simulink model "autopilot_gazebo"  (R2016a)
settings: Solver=ode3  StartTime=0.0  StopTime=30  FixedStep=0.01  RelTol=1e-3
values from neighbouring files (symbols this model uses):
  Kx = KK(:,1:8)    [drone_config.m]
  Ky = KK(:,9:12)    [drone_config.m]
undefined symbols (not defined in the file or in its folder): DiscIntNeverNeededParam, sigbuilder_block, W, X, Y, Z
libraries: simulink_extras x3, robotlib x3, aerolibtransform2 x2, simulink x1
settings Model: Creator=rcasado  LastModifiedBy=rcasado
settings DataIOCC: LimitDataPoints=on  SaveFormat=Array
settings DebuggingCC: MultiTaskRateTransMsg=warning  AllowSymbolicDim=off
settings HardwareCC: ProdBitPerPointer=32  ProdLargestAtomicFloat=None  ProdIntDivRoundTo=Undefined  ProdEndianess=Unspecified  ProdWordSize=32  ProdHWDeviceType=32-bit Generic
settings ModelReferenceCC: PropagateSignalLabelsOutOfModel=off
settings ConfigComp: CovModelRefEnable=Off

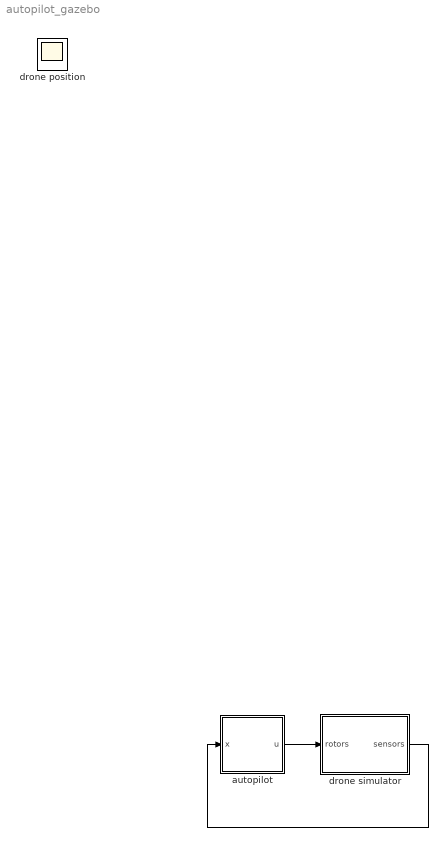
== system autopilot_gazebo ==
  autopilot : Stateflow chart  TreatAsAtomicUnit=on
  drone simulator : Subsystem
  drone position : Scope
  wires:
  drone simulator/1(sensors) -> autopilot/1(x)
  autopilot/1(u) -> drone simulator/1(rotors)

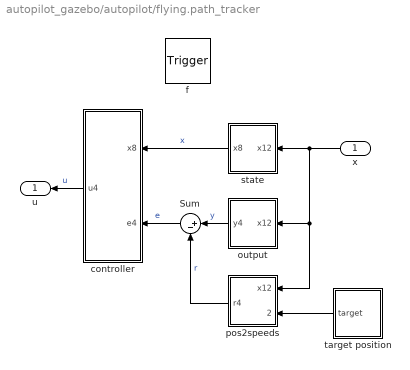
== system autopilot_gazebo/autopilot/flying.path_tracker ==
  x : Inport  OutDataTypeStr=double  PortDimensions=12
  f : TriggerPort  TriggerType=function-call  VariantControl=Variant
      settings: CopyFcn=Stateflow.SLINSF.SimulinkMan.removeBlockPreDeleteFcn  PreDeleteFcn=Stateflow.SLINSF.SimulinkMan.unsafePredeleteFcn
  Sum : Sum  Inputs=|+-
  controller : Subsystem
  output : Subsystem
  pos2speeds : Subsystem
  state : Subsystem
  target position : Subsystem
  u : Outport
  wires:
  x/1 -> pos2speeds/1(x12), output/1(x12), state/1(x12)
  pos2speeds/1(r4) -> Sum/2  "r"
  controller/1(u4) -> u/1  "u"
  output/1(y4) -> Sum/1  "y"
  state/1(x8) -> controller/1(x8)  "x"
  Sum/1 -> controller/2(e4)  "e"
  target position/1(target) -> pos2speeds/2(target)

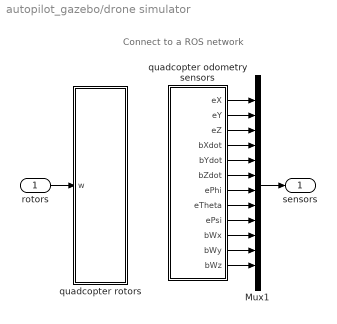
== system autopilot_gazebo/drone simulator ==
  note: Connect to a
      | ROS network
  rotors : Inport
  Mux1 : Mux  Inputs=12
  quadcopter odometry sensors : Subsystem
  quadcopter rotors : Subsystem
  sensors : Outport
  wires:
  quadcopter odometry sensors/1(eX) -> Mux1/1
  rotors/1 -> quadcopter rotors/1(w)
  quadcopter odometry sensors/2(eY) -> Mux1/2
  quadcopter odometry sensors/3(eZ) -> Mux1/3
  Mux1/1 -> sensors/1
  quadcopter odometry sensors/4(bXdot) -> Mux1/4
  quadcopter odometry sensors/5(bYdot) -> Mux1/5
  quadcopter odometry sensors/6(bZdot) -> Mux1/6
  quadcopter odometry sensors/7(ePhi) -> Mux1/7
  quadcopter odometry sensors/8(eTheta) -> Mux1/8
  quadcopter odometry sensors/9(ePsi) -> Mux1/9
  quadcopter odometry sensors/10(bWx) -> Mux1/10
  quadcopter odometry sensors/11(bWy) -> Mux1/11
  quadcopter odometry sensors/12(bWz) -> Mux1/12

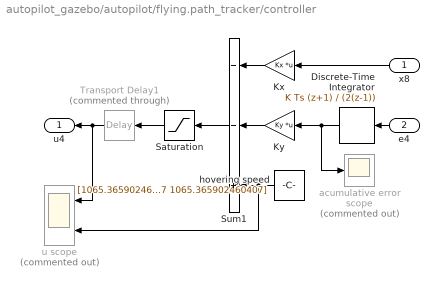
== system autopilot_gazebo/autopilot/flying.path_tracker/controller ==
  x8 : Inport
  e4 : Inport  Port=2
  Discrete-Time Integrator : DiscreteIntegrator  IntegratorMethod=Integration: Trapezoidal  SampleTime=-1  ICPrevOutput=DiscIntNeverNeededParam  ICPrevScaledInput=DiscIntNeverNeededParam
  Kx : Gain  Gain=Kx  Multiplication=Matrix(K*u)
  Ky : Gain  Gain=Ky  Multiplication=Matrix(K*u)
  Saturation : Saturate  UpperLimit=1650  LowerLimit=0
  Sum1 : Sum  Inputs=--+
  Transport Delay1 : TransportDelay  Commented=through  DelayTime=0.05
  acumulative error scope : Scope  Commented=on
  hovering speed : Constant  Value=[1065.365902460407 1065.365902460407 1065.365902460407 1065.365902460407]
  u scope : Scope  Commented=on  NumInputPorts=2
  u4 : Outport
  wires:
  Saturation/1 -> Transport Delay1/1
  Kx/1 -> Sum1/1
  x8/1 -> Kx/1
  hovering speed/1 -> u scope/2, Sum1/3
  Sum1/1 -> Saturation/1
  Transport Delay1/1 -> u scope/1, u4/1
  e4/1 -> Discrete-Time Integrator/1
  Ky/1 -> Sum1/2
  Discrete-Time Integrator/1 -> Ky/1, acumulative error scope/1

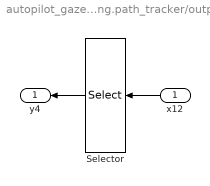
== system autopilot_gazebo/autopilot/flying.path_tracker/output ==
  x12 : Inport
  Selector : Selector  InputPortWidth=12  IndexOptions=Index vector (dialog)  Indices=[4 5 6 12]  OutputSizes=1
  y4 : Outport
  wires:
  x12/1 -> Selector/1
  Selector/1 -> y4/1

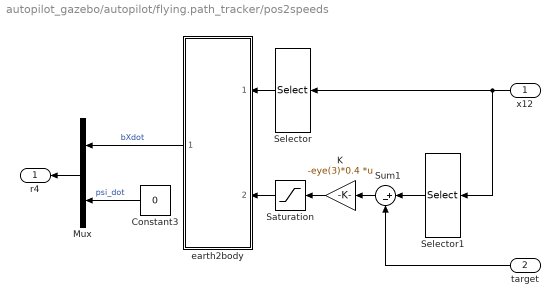
== system autopilot_gazebo/autopilot/flying.path_tracker/pos2speeds ==
  x12 : Inport
  target : Inport  Port=2
  Constant3 : Constant  Value=0
  K : Gain  Gain=-eye(3)*0.4  Multiplication=Matrix(K*u)
  Mux : Mux  Inputs=2
  Saturation : Saturate  UpperLimit=2  LowerLimit=-2
  Selector : Selector  InputPortWidth=12  IndexOptions=Index vector (dialog)  Indices=[7,8,9]  OutputSizes=1
  Selector1 : Selector  InputPortWidth=12  IndexOptions=Index vector (dialog)  Indices=[1;2;3]  OutputSizes=1
  Sum1 : Sum  Inputs=|+-
  earth2body : Subsystem
  r4 : Outport
  wires:
  Mux/1 -> r4/1
  Saturation/1 -> earth2body/2(eXYZdot)
  Constant3/1 -> Mux/2  "psi_dot"
  earth2body/1(bXYZdot) -> Mux/1  "bXdot"
  Selector1/1 -> Sum1/1
  K/1 -> Saturation/1
  Sum1/1 -> K/1
  x12/1 -> Selector1/1, Selector/1
  target/1 -> Sum1/2
  Selector/1 -> earth2body/1(orientation)

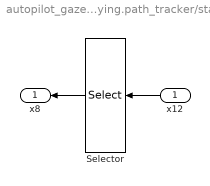
== system autopilot_gazebo/autopilot/flying.path_tracker/state ==
  x12 : Inport
  Selector : Selector  InputPortWidth=12  IndexOptions=Index vector (dialog)  Indices=[7 8 10 11 12 4 5 6]  OutputSizes=1
  x8 : Outport
  wires:
  x12/1 -> Selector/1
  Selector/1 -> x8/1

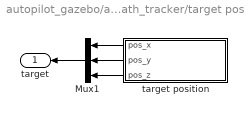
== system autopilot_gazebo/autopilot/flying.path_tracker/target position ==
  Mux1 : Mux  Inputs=3
  target position : Subsystem  Tag=STV Subsys  LoadFcn=sigbuilder_block('load');  StartFcn=sigbuilder_block('start');  StopFcn=sigbuilder_block('stop');  ClipboardFcn=sigbuilder_block('clipboard');  mask(Sigbuilder block){}
      mask help: Simulink:masks:SigbuilderBlock_MD
      mask init:
      | if ~strcmp(get_param(bdroot(gcbh),'SimulationStatus'),'stopped') tuvar = sigbuilder_block('maskInit'); end
      settings: CopyFcn=sigbuilder_block('copy');  DeleteFcn=sigbuilder_block('delete');  ModelCloseFcn=sigbuilder_block('modelClose');  PreSaveFcn=sigbuilder_block('preSave');  PauseFcn=sigbuilder_block('pause');  ContinueFcn=sigbuilder_block('continue');  NameChangeFcn=sigbuilder_block('namechange');  OpenFcn=sigbuilder_block('open',[682.5 614.25 384.75 504 ]);  CloseFcn=sigbuilder_block('close');
      mask Display: plot(0, 0, 100, 100,[2, 2, 32, 32, 2], [68, 8, 8, 68, 68],[32, 2], [38, 38], [32, 19, 2],[53, 60, 44], [32, 17, 17, 2],[16, 16, 31, 31]);txt = getActiveGroup(gcbh);text(2, 100, txt,'verticalAlignment', 'top');
  target : Outport
  wires:
  target position/3(pos_z) -> Mux1/3
  target position/1(pos_x) -> Mux1/1
  target position/2(pos_y) -> Mux1/2
  Mux1/1 -> target/1

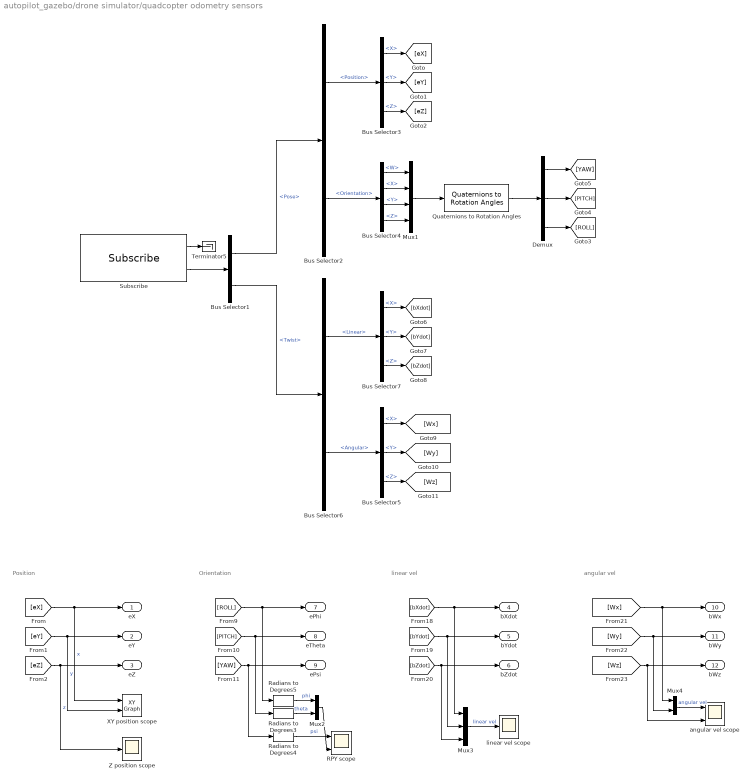
== system autopilot_gazebo/drone simulator/quadcopter odometry sensors ==
  note: linear vel
  note: Position
  note: Orientation
  note: angular vel
  Bus Selector1 : BusSelector  DialogController=Simulink.DDGSource_BusSelector  OutputSignals=Pose,Twist
  Bus Selector2 : BusSelector  DialogController=Simulink.DDGSource_BusSelector  OutputSignals=Position,Orientation
  Bus Selector3 : BusSelector  DialogController=Simulink.DDGSource_BusSelector  OutputSignals=X,Y,Z
  Bus Selector4 : BusSelector  DialogController=Simulink.DDGSource_BusSelector  OutputSignals=W,X,Y,Z
  Bus Selector5 : BusSelector  DialogController=Simulink.DDGSource_BusSelector  OutputSignals=X,Y,Z
  Bus Selector6 : BusSelector  DialogController=Simulink.DDGSource_BusSelector  OutputSignals=Linear,Angular
  Bus Selector7 : BusSelector  DialogController=Simulink.DDGSource_BusSelector  OutputSignals=X,Y,Z
  Demux : Demux  Outputs=3
  Mux1 : Mux
  Mux2 : Mux  Inputs=2
  Mux3 : Mux  Inputs=3
  Mux4 : Mux  Inputs=2
  Quaternions to Rotation Angles : aerolibtransform2/Quaternions to Rotation Angles  rotationOrder=ZYX
  RPY scope : Scope  NumInputPorts=2
  Radians to Degrees3 : simulink_extras/Transformations/Radians to Degrees
  Radians to Degrees4 : simulink_extras/Transformations/Radians to Degrees
  Radians to Degrees5 : simulink_extras/Transformations/Radians to Degrees
  Subscribe : robotlib/Subscribe  SourceLibraryInfo=This block requires Robotics System Toolbox  topicSource=Specify your own  topic=/quadcopter/odometry  messageType=gazebo_msgs/ModelState  sampleTime=-1  messageQueueLength=51
  Terminator5 : Terminator
  XY position scope : simulink/Sinks/XY Graph  xmin=-10  xmax=10  ymin=-10  ymax=10  st=-1
  Z position scope : Scope
  angular vel scope : Scope  NumInputPorts=2
  linear vel scope : Scope
  eX : Outport
  eY : Outport  Port=2
  eZ : Outport  Port=3
  bXdot : Outport  Port=4
  bYdot : Outport  Port=5
  bZdot : Outport  Port=6
  ePhi : Outport  Port=7
  eTheta : Outport  Port=8
  ePsi : Outport  Port=9
  bWx : Outport  Port=10
  bWy : Outport  Port=11
  bWz : Outport  Port=12
  wires:
  Subscribe/2 -> Bus Selector1/1
  Bus Selector1/1 -> Bus Selector2/1  "<Pose>"
  Bus Selector1/2 -> Bus Selector6/1  "<Twist>"
  Subscribe/1 -> Terminator5/1
  Bus Selector2/1 -> Bus Selector3/1  "<Position>"
  Bus Selector3/1 -> [eX]  "<X>"
  Bus Selector3/2 -> [eY]  "<Y>"
  Bus Selector3/3 -> [eZ]  "<Z>"
  [eX] -> XY position scope/1, eX/1  "x"
  [eY] -> XY position scope/2, eY/1  "y"
  [eZ] -> Z position scope/1, eZ/1  "z"
  Bus Selector2/2 -> Bus Selector4/1  "<Orientation>"
  Quaternions to Rotation Angles/1 -> Demux/1
  [PITCH] -> eTheta/1, Radians to Degrees3/1
  [ROLL] -> ePhi/1, Radians to Degrees5/1
  Demux/1 -> [YAW]
  Demux/3 -> [ROLL]
  Demux/2 -> [PITCH]
  Mux1/1 -> Quaternions to Rotation Angles/1
  Bus Selector4/1 -> Mux1/1  "<W>"
  Bus Selector4/2 -> Mux1/2  "<X>"
  Bus Selector4/3 -> Mux1/3  "<Y>"
  Bus Selector4/4 -> Mux1/4  "<Z>"
  Bus Selector6/1 -> Bus Selector7/1  "<Linear>"
  Bus Selector7/1 -> [bXdot]  "<X>"
  Bus Selector7/2 -> [bYdot]  "<Y>"
  Bus Selector7/3 -> [bZdot]  "<Z>"
  Bus Selector6/2 -> Bus Selector5/1  "<Angular>"
  Bus Selector5/1 -> [Wx]  "<X>"
  Bus Selector5/2 -> [Wy]  "<Y>"
  Bus Selector5/3 -> [Wz]  "<Z>"
  Mux3/1 -> linear vel scope/1  "linear vel"
  Mux4/1 -> angular vel scope/1  "angular vel"
  [Wx] -> bWx/1, Mux4/1
  [Wy] -> bWy/1, Mux4/2
  [Wz] -> angular vel scope/2, bWz/1
  [bXdot] -> Mux3/1, bXdot/1
  [bYdot] -> Mux3/2, bYdot/1
  [bZdot] -> Mux3/3, bZdot/1
  [YAW] -> Radians to Degrees4/1, ePsi/1
  Radians to Degrees3/1 -> Mux2/2  "theta"
  Radians to Degrees4/1 -> RPY scope/1  "psi"
  Radians to Degrees5/1 -> Mux2/1  "phi"
  Mux2/1 -> RPY scope/2

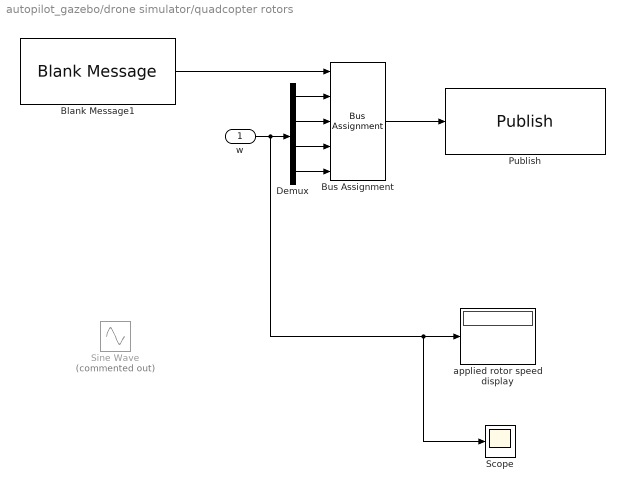
== system autopilot_gazebo/drone simulator/quadcopter rotors ==
  w : Inport
  Blank Message1 : robotlib/Blank Message  SourceLibraryInfo=This block requires Robotics System Toolbox  messageType=geometry_msgs/Quaternion  SampleTime=0.01
  Bus Assignment : BusAssignment  AssignedSignals=X,Y,Z,W
  Demux : Demux
  Publish : robotlib/Publish  SourceLibraryInfo=This block requires Robotics System Toolbox  topicSource=Select from ROS network  topic=/quadcopter/rotor_speeds  messageType=geometry_msgs/Quaternion  messageQueueLength=105
  Scope : Scope
  Sine Wave : Sin  Commented=on  Amplitude=500  Bias=1000  Frequency=2*pi/10  Phase=-pi/2  SampleTime=0
  applied rotor speed display : Display
      settings: Decimation=5
  wires:
  Bus Assignment/1 -> Publish/1
  w/1 -> Scope/1, applied rotor speed display/1, Demux/1
  Blank Message1/1 -> Bus Assignment/1
  Demux/4 -> Bus Assignment/5
  Demux/3 -> Bus Assignment/4
  Demux/2 -> Bus Assignment/3
  Demux/1 -> Bus Assignment/2

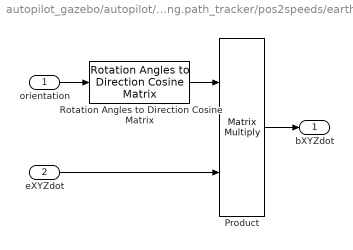
== system autopilot_gazebo/autopilot/flying.path_tracker/pos2speeds/earth2body ==
  orientation : Inport
  eXYZdot : Inport  Port=2
  Product : Product  Multiplication=Matrix(*)
  Rotation Angles to Direction Cosine Matrix : aerolibtransform2/Rotation Angles to Direction Cosine Matrix  rotationOrder=XYZ
  bXYZdot : Outport
  wires:
  Product/1 -> bXYZdot/1
  Rotation Angles to Direction Cosine Matrix/1 -> Product/1
  eXYZdot/1 -> Product/2
  orientation/1 -> Rotation Angles to Direction Cosine Matrix/1

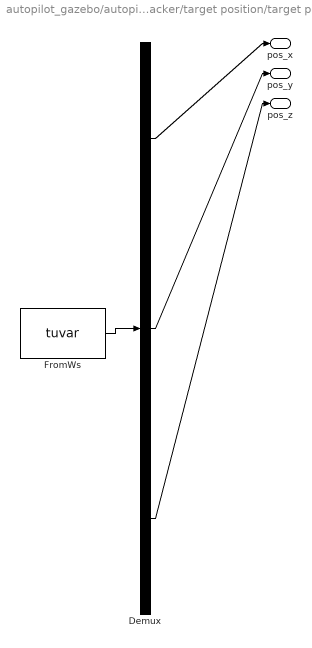
== system autopilot_gazebo/autopilot/flying.path_tracker/target position/target position ==
  Demux : Demux  Tag=STV Demux  Outputs=3
  FromWs : FromWorkspace  Tag=STV FromWs  VariableName=tuvar  OutputAfterFinalValue=Setting to zero
      SigBuilderData=|
      | common.afterFinalStr = 'Set to zero'
      | common.sampleTime = '-1'
      | dataSet(1).timeRange = [0 20]
      | dataSet(1).name = 've y aterriza'
      | dataSet(2).timeRange = [0 10]
      | dataSet(2).name = 'avanza1'
      | sbobj.Groups(1).Name = 've y aterriza'
      | sbobj.Groups(1).Signals(1).Name = 'pos_x'
      | sbobj.Groups(1).Signals(1).XData = [0 1 5 20]
      | sbobj.Groups(1).Signals(1).YData = [0 0 6 6]
      | sbobj.Groups(1).Signals(2).Name = 'pos_y'
      | sbobj.Groups(1).Signals(2).XData = [0 1 5 20]
      | sbobj.Groups(1).Signals(2).YData = [0 0 3 3]
      | sbobj.Groups(1).Signals(3).Name = 'pos_z'
      | sbobj.Groups(1).Signals(3).XData = [0 2 10 13 15 20]
      | sbobj.Groups(1).Signals(3).YData = [0 4 4 1 0 0]
      | sbobj.Groups(1).TimeRange = [0 20]
      | sbobj.Groups(2).Name = 'avanza1'
      | sbobj.Groups(2).Signals(1).Name = 'pos_x'
      | sbobj.Groups(2).Signals(1).XData = [0 1 1 4 6 10]
      | sbobj.Groups(2).Signals(1).YData = [0 0 3 3 3 3]
      | sbobj.Groups(2).Signals(2).Name = 'pos_y'
      | sbobj.Groups(2).Signals(2).XData = [0 4 10]
      | sbobj.Groups(2).Signals(2).YData = [0 4 4]
      | sbobj.Groups(2).Signals(3).Name = 'pos_z'
      | sbobj.Groups(2).Signals(3).XData = [0 6 6 10]
      | sbobj.Groups(2).Signals(3).YData = [10 10 0 0]
  pos_x : Outport  Tag=STV Outport
  pos_y : Outport  Tag=STV Outport  Port=2
  pos_z : Outport  Tag=STV Outport  Port=3
  wires:
  FromWs/1 -> Demux/1
  Demux/1 -> pos_x/1
  Demux/2 -> pos_y/1
  Demux/3 -> pos_z/1

== stateflow chart autopilot_gazebo/autopilot ==
  settings: updateMethod=DISCRETE  sampleTime=0.01  executeAtInitialization=1
  state take_off
    during:
    u = [0; 0; 0; 0];
  state flying
    during:
    u = path_tracker(x);
    state u = path_tracker(x) [function]
  state landing
    during:
    u = [0; 0; 0; 0];
  (default) -> take_off
  take_off -> flying
  flying -> landing : after(20,sec)
  data: u function_output; x function_input double size=12; x input size=12; u output size=4
